simulink model "cascadedmultilevelinverter"  (Simulink 7.5)
settings: Solver=ode23tb  StartTime=0.0  StopTime=0.1  MaxStep=1e-5  RelTol=1e-3
libraries: powerlib x18, simulink x4
settings Model: Creator=viswam  LastModifiedBy=placements
settings SolverCC: InitialStep=1e-6
settings OptimizationCC: InitFltsAndDblsToZero=on
settings DebuggingCC: SaveWithParameterizedLinksMsg=none  SignalResolutionControl=TryResolveAllWithWarning  MultiTaskDSMMsg=warning  MultiTaskCondExecSysMsg=none  StrictBusMsg=Warning
settings RTWCC: IncludeERTFirstTime=on
settings GRTTargetCC: TargetFcnLib=ansi_tfl_tmw.mat

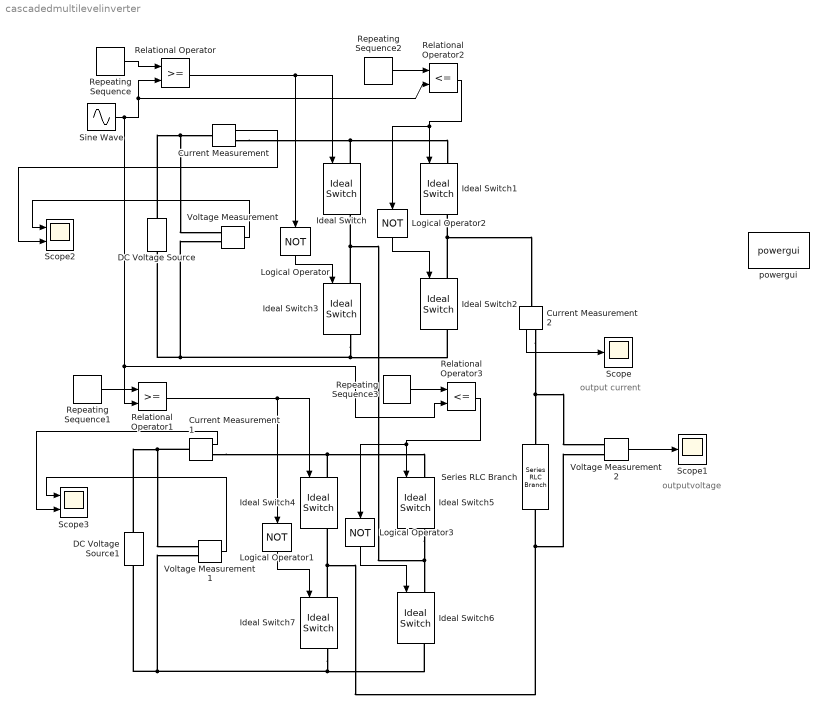
== system cascadedmultilevelinverter ==
  note: output current
  note: outputvoltage
  Current Measurement : powerlib/Measurements/Current Measurement  DialogController=POWERSYS.PowerSysDialog  SystemSampleTime=-1  PhasorSimulation=off  OutputType=Complex  PSBequivalent=0
  Current Measurement1 : powerlib/Measurements/Current Measurement  DialogController=POWERSYS.PowerSysDialog  SystemSampleTime=-1  PhasorSimulation=off  OutputType=Complex  PSBequivalent=0
  Current Measurement2 : powerlib/Measurements/Current Measurement  DialogController=POWERSYS.PowerSysDialog  SystemSampleTime=-1  PhasorSimulation=off  OutputType=Complex  PSBequivalent=0
  DC Voltage Source : powerlib/Electrical Sources/DC Voltage Source  DialogController=POWERSYS.PowerSysDialog  SystemSampleTime=-1  Amplitude=100  Measurements=None
  DC Voltage Source1 : powerlib/Electrical Sources/DC Voltage Source  DialogController=POWERSYS.PowerSysDialog  SystemSampleTime=-1  Amplitude=100  Measurements=None
  Ideal Switch{,1..7} (8 alike) : powerlib/Power Electronics/Ideal Switch  DialogController=POWERSYS.PowerSysDialog  SystemSampleTime=-1  Ron=0.001  Lon=0  IC=0  Rs=1e5  Cs=inf  Measurements=on
  Logical Operator{,1..3} (4 alike) : Logic  Operator=NOT  AllPortsSameDT=off  OutDataTypeMode=boolean  OutDataTypeStr=boolean
  Relational Operator : RelationalOperator  LogicOutDataTypeMode=boolean  OutDataTypeStr=boolean
  Relational Operator1 : RelationalOperator  LogicOutDataTypeMode=boolean  OutDataTypeStr=boolean
  Relational Operator2 : RelationalOperator  Operator=<=  LogicOutDataTypeMode=boolean  OutDataTypeStr=boolean
  Relational Operator3 : RelationalOperator  Operator=<=  LogicOutDataTypeMode=boolean  OutDataTypeStr=boolean
  Repeating Sequence : simulink/Sources/Repeating Sequence  SystemSampleTime=-1  rep_seq_t=[0 0.5e-3 1e-3]  rep_seq_y=[0 1/2 0]
  Repeating Sequence1 : simulink/Sources/Repeating Sequence  SystemSampleTime=-1  rep_seq_t=[0 0.5e-3 1e-3]  rep_seq_y=[1/2 1 1/2]
  Repeating Sequence2 : simulink/Sources/Repeating Sequence  SystemSampleTime=-1  rep_seq_t=[0 0.5e-3 1e-3]  rep_seq_y=[-1/2 0 -1/2]
  Repeating Sequence3 : simulink/Sources/Repeating Sequence  SystemSampleTime=-1  rep_seq_t=[0 0.5e-3 1e-3]  rep_seq_y=[-1 -1/2 -1]
  Scope : Scope
      settings: SaveName=outputcurrent
  Scope1 : Scope
      settings: SaveName=outputvoltage
  Scope2 : Scope  NumInputPorts=2
      settings: YMin=-5~-5  YMax=5~5  SaveName=outputvoltage1
  Scope3 : Scope  NumInputPorts=2
      settings: YMin=-5~-5  YMax=5~5  SaveName=outputvoltage2
  Series RLC Branch : powerlib/Elements/Series RLC Branch  DialogController=POWERSYS.PowerSysDialog  PhysicalDomain=powersysdomain  SubClassName=unknown  LeftPortType=p1  RightPortType=p1  LConnTagsString=__new0  RConnTagsString=__new0  BranchType=R  Resistance=10  Inductance=1e-3  SetiL0=off  InitialCurrent=0  Capacitance=1e-6  Setx0=off  InitialVoltage=0  Measurements=None
  Sine Wave : Sin  Amplitude=1  Bias=0  Frequency=2*pi*50  Phase=0  Samples=10  SampleTime=0  Offset=0
  Voltage Measurement : powerlib/Measurements/Voltage Measurement  DialogController=POWERSYS.PowerSysDialog  SystemSampleTime=-1  PhasorSimulation=off  OutputType=Complex  PSBequivalent=0
  Voltage Measurement1 : powerlib/Measurements/Voltage Measurement  DialogController=POWERSYS.PowerSysDialog  SystemSampleTime=-1  PhasorSimulation=off  OutputType=Complex  PSBequivalent=0
  Voltage Measurement2 : powerlib/Measurements/Voltage Measurement  DialogController=POWERSYS.PowerSysDialog  SystemSampleTime=-1  PhasorSimulation=off  OutputType=Complex  PSBequivalent=0
  powergui : powerlib/powergui  Priority=1  SystemSampleTime=-1  SimulationMode=Continuous  SampleTime=50e-6  frequency=60  SPID=off  DisableSnubberDevices=off  DisableRonSwitches=off  DisableVfSwitches=off  SwTol=0  Interpol=off  frequencyindice=0  echomessages=off  HookPort=off  DisplayEquations=off  FunctionMessages=off  EnableUseOfTLC=off  x0status=blocks  RestoreLinks=warning  ResistiveCurrentMeasurement=off  Frange=[0:2:500]  Ylog=off  Xlog=on  ShowGrid=off  save=off  variable=ZData  structure=outputvoltage  ZoomFFT=off  StartTime=0.0  cycles=1  DisplayStyle=1  fundamental=50  FreqAxis=on  MaxFrequency=1000  frequencyindicesteady=1  RmsSteady=1  display=off  Ts=0  methode=off
  wires:
  Repeating Sequence/1 -> Relational Operator/1
  Sine Wave/1 -> Relational Operator/2, Relational Operator2/2, Relational Operator1/2, Relational Operator3/2
  Relational Operator/1 -> Ideal Switch/1, Logical Operator/1
  Logical Operator/1 -> Ideal Switch3/1
  Repeating Sequence1/1 -> Relational Operator1/1
  Relational Operator1/1 -> Ideal Switch4/1, Logical Operator1/1
  Logical Operator1/1 -> Ideal Switch7/1
  Repeating Sequence2/1 -> Relational Operator2/1
  Relational Operator2/1 -> Ideal Switch1/1, Logical Operator2/1
  Logical Operator2/1 -> Ideal Switch2/1
  Repeating Sequence3/1 -> Relational Operator3/1
  Relational Operator3/1 -> Ideal Switch5/1, Logical Operator3/1
  Logical Operator3/1 -> Ideal Switch6/1
  Current Measurement2/1 -> Scope/1
  Voltage Measurement2/1 -> Scope1/1
  Voltage Measurement/1 -> Scope2/1
  Current Measurement/1 -> Scope2/2
  Voltage Measurement1/1 -> Scope3/1
  Current Measurement1/1 -> Scope3/2
  connections:
  Ideal Switch2/LConn1 -- Ideal Switch1/RConn1 -- Current Measurement2/LConn1
  Ideal Switch3/RConn1 -- Ideal Switch2/RConn1 -- DC Voltage Source/LConn1 -- Voltage Measurement/LConn2
  Ideal Switch/LConn1 -- Ideal Switch1/LConn1 -- Current Measurement/RConn1
  DC Voltage Source/RConn1 -- Current Measurement/LConn1 -- Voltage Measurement/LConn1
  Ideal Switch6/RConn1 -- Ideal Switch7/RConn1 -- Voltage Measurement1/LConn2 -- DC Voltage Source1/LConn1
  Ideal Switch4/LConn1 -- Current Measurement1/RConn1 -- Ideal Switch5/LConn1
  Current Measurement1/LConn1 -- Voltage Measurement1/LConn1 -- DC Voltage Source1/RConn1
  Ideal Switch7/LConn1 -- Ideal Switch4/RConn1 -- Series RLC Branch/RConn1 -- Voltage Measurement2/LConn2
  Ideal Switch5/RConn1 -- Ideal Switch6/LConn1 -- Ideal Switch3/LConn1 -- Ideal Switch/RConn1
  Current Measurement2/RConn1 -- Series RLC Branch/LConn1 -- Voltage Measurement2/LConn1
